simulink model "GVCU_HIL"  (R2026a)
settings: Solver=ode3  StartTime=0  StopTime=2474  FixedStep=0.0002
model workspace (MAT data in the model file):
  CANoelibParameters : object (value not decoded)
values from neighbouring files (symbols this model uses):
  acc_pedal_data = pedal_data.accelerator_pedal_position_t0    [Vehicle_Simulink_init.m]
  acc_pedal_time = pedal_data.t0    [Vehicle_Simulink_init.m]
  brk_pedal_data = brake_pedal_data.shared_brakes_drvrBrkPedlPerc_t0    [Vehicle_Simulink_init.m]
  brk_pedal_time = brake_pedal_data.t0    [Vehicle_Simulink_init.m]
  cycle_len = zeros(1, num_cycles)    [Vehicle_Simulink_init.m]
  cycle_speed_matrix = zeros(max_cycle_len, num_cycles)    [Vehicle_Simulink_init.m]
  cycle_time_matrix = zeros(max_cycle_len, num_cycles)    [Vehicle_Simulink_init.m]
  veh_speed_data = speed_data.shared_dynamicsVso_vehVelLgt_t0    [Vehicle_Simulink_init.m]
  veh_speed_time = speed_data.t0    [Vehicle_Simulink_init.m]
undefined symbols (not defined in the file or in its folder): Active, AuxActive, bat, environment, FL_prs_voltage, FR_prs_voltage, pos, RL_prs_voltage, RR_prs_voltage, tir, veh, VGetRawValueFlag, Voltage, VT2816_1_Ch1, VT2816_1_Ch2, VT2816_1_Ch3, VT2816_1_Ch4, VT2816_3_Ch13, VT2816_3_Ch14, VT7101_1_Out2, VT7820_2_Channel1, VT7820_2_Channel2, VT7820_2_Channel3, VT7820_2_Channel4, VTS
libraries: canoelib x144, autolibsharedcoupling x21, autolibcoupling x9, autolibshared x5, simulink_extras x4, simulink x4, slpidlib x3, autolibshareddiff x3, autolibutils x1, autolibdatasheetbattery x1, autolibmappedmotor x1, sl_discontinuities x1
(part 8 of 9)

== system GVCU_HIL/Vehicle/to grade ==
  In1 : Inport
  Constant : Constant  Value=veh.f + veh.r
  Divide : Product  Inputs=*/
  Gain : Gain  Gain=0.5
  Gain1 : Gain  Gain=0.5
  "Radians to Degrees " : simulink_extras/Transformations/Radians to Degrees
  Selector : Selector  InputPortWidth=4  IndexOptions=Index vector (dialog)  Indices=[1]  OutputSizes=1
  Selector1 : Selector  InputPortWidth=4  IndexOptions=Index vector (dialog)  Indices=[2]  OutputSizes=1
  Selector2 : Selector  InputPortWidth=4  IndexOptions=Index vector (dialog)  Indices=[3]  OutputSizes=1
  Selector3 : Selector  InputPortWidth=4  IndexOptions=Index vector (dialog)  Indices=[4]  OutputSizes=1
  Sum : Sum
  Sum1 : Sum
  Sum2 : Sum  Inputs=+-
  "Tan " : Trigonometry  Operator=asin
  Out1 : Outport
  wires:
  "Radians to Degrees "/1 -> Out1/1
  "Tan "/1 -> "Radians to Degrees "/1
  Divide/1 -> "Tan "/1
  Constant/1 -> Divide/2
  Sum2/1 -> Divide/1
  Gain1/1 -> Sum2/2
  Gain/1 -> Sum2/1
  Sum1/1 -> Gain1/1
  Sum/1 -> Gain/1
  Selector3/1 -> Sum1/2
  Selector2/1 -> Sum1/1
  Selector1/1 -> Sum/2
  Selector/1 -> Sum/1
  In1/1 -> Selector/1, Selector1/1, Selector2/1, Selector3/1

== system GVCU_HIL/Brake_HIL/Simulated GVCU - Steering /Message Output ==
  In1 : Inport
  Bus Selector : BusSelector  OutputSignals=drv_mod,e2e_alive_counter,e2e_checksum,hhc_inhb_req,ieb_chg_mod_req,vdc_perf_mod_req
  S-Function_1 : S-Function  FunctionName=sigout  Parameters=dbName;nodeName;msgName;6;'drv_mod';'e2e_alive_counter';'e2e_checksum';'hhc_inhb_req';'ieb_chg_mod_req';'vdc_perf_mod_req';VGetRawValueFlag(rawValue);'inherited'  SFunctionDeploymentMode=off  EnableBusSupport=off
      settings: AttributesFormatString=drv_mod\ne2e_alive_counter\ne2e_checksum\nhhc_inhb_req\nieb_chg_mod_req\nvdc_perf_mod_req\n
  wires:
  Bus Selector/5 -> S-Function_1/5  "<ieb_chg_mod_req>"
  Bus Selector/4 -> S-Function_1/4  "<hhc_inhb_req>"
  Bus Selector/3 -> S-Function_1/3  "<e2e_checksum>"
  Bus Selector/2 -> S-Function_1/2  "<e2e_alive_counter>"
  Bus Selector/1 -> S-Function_1/1  "<drv_mod>"
  In1/1 -> Bus Selector/1
  Bus Selector/6 -> S-Function_1/6  "<vdc_perf_mod_req>"

== system GVCU_HIL/Brake_HIL/Simulated GVCU - Steering /Message Output1 ==
  In1 : Inport
  Bus Selector : BusSelector  OutputSignals=e2e_alive_counter,e2e_checksum,lat_acc,lat_acc_v,long_acc,long_acc_v,yaw_rate,yaw_rate_v
  S-Function_1 : S-Function  FunctionName=sigout  Parameters=dbName;nodeName;msgName;8;'e2e_alive_counter';'e2e_checksum';'lat_acc';'lat_acc_v';'long_acc';'long_acc_v';'yaw_rate';'yaw_rate_v';VGetRawValueFlag(rawValue);'inherited'  SFunctionDeploymentMode=off  EnableBusSupport=off
      settings: AttributesFormatString=e2e_alive_counter\ne2e_checksum\nlat_acc\nlat_acc_v\nlong_acc\nlong_acc_v\nyaw_rate\nyaw_rate_v\n
  wires:
  Bus Selector/8 -> S-Function_1/8  "<yaw_rate_v>"
  Bus Selector/7 -> S-Function_1/7  "<yaw_rate>"
  Bus Selector/6 -> S-Function_1/6  "<long_acc_v>"
  Bus Selector/5 -> S-Function_1/5  "<long_acc>"
  Bus Selector/4 -> S-Function_1/4  "<lat_acc_v>"
  Bus Selector/3 -> S-Function_1/3  "<lat_acc>"
  Bus Selector/2 -> S-Function_1/2  "<e2e_checksum>"
  Bus Selector/1 -> S-Function_1/1  "<e2e_alive_counter>"
  In1/1 -> Bus Selector/1

== system GVCU_HIL/Brake_HIL/Simulated GVCU - Steering /Message Output2 ==
  In1 : Inport
  Bus Selector : BusSelector  OutputSignals=calibration_sts,e2e_alive_counter,e2e_checksum,steering_wheel_angle,steering_wheel_rot_speed,steering_wheel_sensor_v
  S-Function_1 : S-Function  FunctionName=sigout  Parameters=dbName;nodeName;msgName;6;'calibration_sts';'e2e_alive_counter';'e2e_checksum';'steering_wheel_angle';'steering_wheel_rot_speed';'steering_wheel_sensor_v';VGetRawValueFlag(rawValue);'inherited'  SFunctionDeploymentMode=off  EnableBusSupport=off
      settings: AttributesFormatString=calibration_sts\ne2e_alive_counter\ne2e_checksum\nsteering_wheel_angle\nsteering_wheel_rot_speed\nsteering_wheel_sensor_v\n
  wires:
  Bus Selector/6 -> S-Function_1/6  "<steering_wheel_sensor_v>"
  Bus Selector/5 -> S-Function_1/5  "<steering_wheel_rot_speed>"
  Bus Selector/4 -> S-Function_1/4  "<steering_wheel_angle>"
  Bus Selector/3 -> S-Function_1/3  "<e2e_checksum>"
  Bus Selector/2 -> S-Function_1/2  "<e2e_alive_counter>"
  Bus Selector/1 -> S-Function_1/1  "<calibration_sts>"
  In1/1 -> Bus Selector/1

== system GVCU_HIL/Brake_HIL/Simulated GVCU - Steering /Message Output3 ==
  In1 : Inport
  Bus Selector : BusSelector  OutputSignals=e2e_alive_counter,e2e_checksum,nm_request
  S-Function_1 : S-Function  FunctionName=sigout  Parameters=dbName;nodeName;msgName;3;'e2e_alive_counter';'e2e_checksum';'nm_request';VGetRawValueFlag(rawValue);'inherited'  SFunctionDeploymentMode=off  EnableBusSupport=off
      settings: AttributesFormatString=e2e_alive_counter\ne2e_checksum\nnm_request\n
  wires:
  Bus Selector/3 -> S-Function_1/3  "<nm_request>"
  Bus Selector/2 -> S-Function_1/2  "<e2e_checksum>"
  Bus Selector/1 -> S-Function_1/1  "<e2e_alive_counter>"
  In1/1 -> Bus Selector/1

== system GVCU_HIL/Driver/Driver/Dec_controller ==
  Vel_ref : Inport
  Vel_fdk : Inport  Port=2
  PI Controller : slpidlib/PID Controller  Controller=PI  Form=Parallel  TimeDomain=Discrete-time  UseExternalTs=off  SampleTime=-1  IntegratorMethod=Forward Euler  FilterMethod=Forward Euler  ControllerParametersSource=internal  P=1  I=1  UseKiTs=on  D=0  UseExternalDerivativeSource=off  N=100  UseFilter=on  TunerSelectOption=Transfer Function Based (PID Tuner App)  InitialConditionSource=internal  InitialConditionForIntegrator=0  InitialConditionForFilter=0  DifferentiatorICPrevScaledInput=0  ExternalReset=level  TrackingMode=off  Kt=1  LimitOutput=on  SatLimitsSource=internal  UpperSaturationLimit=50  LowerSaturationLimit=0  LinearizeAsGain=on  AntiWindupMode=clamping  Kb=1  LimitIntegrator=off  UpperIntegratorSaturationLimit=inf  LowerIntegratorSaturationLimit=-inf  RndMeth=Simplest  POutMin=[]  POutMax=[]  IOutMin=[]  IOutMax=[]  DOutMin=[]  DOutMax=[]  NOutMin=[]  NOutMax=[]  SumOutMin=[]  SumOutMax=[]  SaturationOutDataTypeStr=Inherit: Inherit via back propagation  SaturationOutMin=[]  SaturationOutMax=[]  PParamMin=[]  PParamMax=[]  IParamMin=[]  IParamMax=[]  DParamMin=[]  DParamMax=[]  NParamMin=[]  NParamMax=[]  KbParamMin=[]  KbParamMax=[]  KtParamMin=[]  KtParamMax=[]  KbOutMin=[]  KbOutMax=[]  KtOutMin=[]  KtOutMax=[]  IntegratorOutMin=[]  IntegratorOutMax=[]  FilterOutMin=[]  FilterOutMax=[]  SumI1OutMin=[]  SumI1OutMax=[]  SumI2OutMin=[]  SumI2OutMax=[]  SumI3OutMin=[]  SumI3OutMax=[]  SumI4OutMin=[]  SumI4OutMax=[]  SumDOutMin=[]  SumDOutMax=[]  DifferentiatorOutMin=[]  DifferentiatorOutMax=[]  FilterDiffOutCoefMin=[]  FilterDiffOutCoefMax=[]  ReciprocalOutMin=[]  ReciprocalOutMax=[]  SumDenOutMin=[]  SumDenOutMax=[]  SumNumOutMin=[]  SumNumOutMax=[]  DivideOutMin=[]  DivideOutMax=[]  UdiffTsProdOutMin=[]  UdiffTsProdOutMax=[]  NTsProdOutMin=[]  NTsProdOutMax=[]  UintegralTsProdOutMin=[]  UintegralTsProdOutMax=[]  UngainTsProdOutMin=[]  UngainTsProdOutMax=[]  ClampingZeroOutDataTypeStr=Inherit: Inherit via back propagation  ClampingZeroOutMin=[]  ClampingZeroOutMax=[]  FilterDenConstantOutDataTypeStr=Inherit: Inherit via back propagation  FilterDenConstantOutMin=[]  FilterDenConstantOutMax=[]  PCopyOutDataTypeStr=Inherit: Inherit via back propagation  PCopyOutMin=[]  PCopyOutMax=[]  NCopyOutDataTypeStr=Inherit: Inherit via back propagation  NCopyOutMin=[]  NCopyOutMax=[]  IntegratorContinuousStateAttributes=''  IntegratorStateMustResolveToSignalObject=off  IntegratorRTWStateStorageClass=Auto  FilterContinuousStateAttributes=''  FilterStateMustResolveToSignalObject=off  FilterRTWStateStorageClass=Auto  ParallelPVariant=InternalParameters  IdealPVariant=Disabled  IVariant=InternalParameters  DVariant=Disabled  IntegratorVariant=Discrete  SatVariant=Enabled  AWVariant=DiscClampingParallel  PCopyVariant=Disabled  TRVariant=Disabled  FdbkBlocksVariant=Forward  IdealPFdbkVariant=Disabled  SatFdbkVariant=Disabled  DerivativeFilterVariant=Disabled  NVariant=Disabled  NCopyVariant=Disabled_SignalSpec  FilterICVariant=Disabled  IntegratorICVariant=InternalICs  ExternalResetVariant=ExternalReset  TRSumVariant=Passthrough  SumFdbkVariant=Disabled  SumVariant=Sum_PI  TsampFilterVariant=InternalTs  TsampNgainVariant=Passthrough  TsampIntegralVariant=Disabled_SignalSpec  ExternalSaturationOutDataTypeStr=Inherit: Same as second input  DerivativeSourceVariant=Disabled  PreIntVariant=InternalPreInt
      settings: LibrarySourceBlock=mcbhdllib/Controls/Controllers/PI Controller
  Relay : Relay  OnSwitchValue=10  OffSwitchValue=1
  Subtract : Sum  Inputs=+-
  Dec_cmd : Outport
  wires:
  Vel_ref/1 -> Subtract/2
  Vel_fdk/1 -> Subtract/1
  PI Controller/1 -> Dec_cmd/1
  Subtract/1 -> PI Controller/1, Relay/1
  Relay/1 -> PI Controller/2

== system GVCU_HIL/Driver/Driver/LPF ==
  u : Inport
  Divide : Product  Inputs=/
  Error LPF : autolibutils/Cont LPF Dyn  aMode=aMode  dataType=off
  tauerr : Constant  Value=0.03  SampleTime=-1
  y : Outport  VectorParamsAs1DForOutWhenUnconnected=off
  wires:
  Error LPF/1 -> y/1
  Divide/1 -> Error LPF/2
  tauerr/1 -> Divide/1
  u/1 -> Error LPF/1

== system GVCU_HIL/GVCU - HiL/Commented messages/Message Output12 ==
  In1 : Inport
  Bus Selector : BusSelector  OutputSignals=e2e_alive_counter_disabled,e2e_checksum_disabled,e_motor_pump_fault,e_motor_pump_power_on,e_motor_pump_speed,e_motor_pump_warning,front_left_fan_fault,front_left_fan_power_on,front_left_fan_speed,front_left_fan_warning,hv_bat_pump_fault,hv_bat_pump_power_on,hv_bat_pump_speed,hv_bat_pump_warning
  S-Function_1 : S-Function  FunctionName=sigout  Parameters=dbName;nodeName;msgName;14;'e2e_alive_counter_disabled';'e2e_checksum_disabled';'e_motor_pump_fault';'e_motor_pump_power_on';'e_motor_pump_speed';'e_motor_pump_warning';'front_left_fan_fault';'front_left_fan_power_on';'front_left_fan_speed';'front_left_fan_warning';'hv_bat_pump_fault';'hv_bat_pump_power_on';'hv_bat_pump_speed';'hv_bat_pump_warning';VGetRawValueFlag(rawValue);'inherited'  SFunctionDeploymentMode=off  EnableBusSupport=off
      settings: AttributesFormatString=e2e_alive_counter_disabled\ne2e_checksum_disabled\ne_motor_pump_fault\ne_motor_pump_power_on\ne_motor_pump_speed\ne_motor_pump_warning\nfront_left_fan_fault\nfront_left_fan_power_on\nfront_left_fan_speed\nfront_left_fan_warning\nhv_bat_pump_fault\nhv_bat_pump_power_on\nhv_bat_pump_speed\nhv_bat_pump_warning\n
  wires:
  In1/1 -> Bus Selector/1
  Bus Selector/1 -> S-Function_1/1  "<e2e_alive_counter_disabled>"
  Bus Selector/2 -> S-Function_1/2  "<e2e_checksum_disabled>"
  Bus Selector/3 -> S-Function_1/3  "<e_motor_pump_fault>"
  Bus Selector/4 -> S-Function_1/4  "<e_motor_pump_power_on>"
  Bus Selector/5 -> S-Function_1/5  "<e_motor_pump_speed>"
  Bus Selector/6 -> S-Function_1/6  "<e_motor_pump_warning>"
  Bus Selector/7 -> S-Function_1/7  "<front_left_fan_fault>"
  Bus Selector/8 -> S-Function_1/8  "<front_left_fan_power_on>"
  Bus Selector/9 -> S-Function_1/9  "<front_left_fan_speed>"
  Bus Selector/10 -> S-Function_1/10  "<front_left_fan_warning>"
  Bus Selector/11 -> S-Function_1/11  "<hv_bat_pump_fault>"
  Bus Selector/12 -> S-Function_1/12  "<hv_bat_pump_power_on>"
  Bus Selector/13 -> S-Function_1/13  "<hv_bat_pump_speed>"
  Bus Selector/14 -> S-Function_1/14  "<hv_bat_pump_warning>"

== system GVCU_HIL/GVCU - HiL/Commented messages/Message Output13 ==
  In1 : Inport
  Bus Selector : BusSelector  OutputSignals=e2e_alive_counter_disabled,e2e_checksum_disabled,inverter_pump_fault,inverter_pump_power_on,inverter_pump_speed,inverter_pump_warning
  S-Function_1 : S-Function  FunctionName=sigout  Parameters=dbName;nodeName;msgName;6;'e2e_alive_counter_disabled';'e2e_checksum_disabled';'inverter_pump_fault';'inverter_pump_power_on';'inverter_pump_speed';'inverter_pump_warning';VGetRawValueFlag(rawValue);'inherited'  SFunctionDeploymentMode=off  EnableBusSupport=off
      settings: AttributesFormatString=e2e_alive_counter_disabled\ne2e_checksum_disabled\ninverter_pump_fault\ninverter_pump_power_on\ninverter_pump_speed\ninverter_pump_warning\n
  wires:
  In1/1 -> Bus Selector/1
  Bus Selector/1 -> S-Function_1/1  "<e2e_alive_counter_disabled>"
  Bus Selector/2 -> S-Function_1/2  "<e2e_checksum_disabled>"
  Bus Selector/3 -> S-Function_1/3  "<inverter_pump_fault>"
  Bus Selector/4 -> S-Function_1/4  "<inverter_pump_power_on>"
  Bus Selector/5 -> S-Function_1/5  "<inverter_pump_speed>"
  Bus Selector/6 -> S-Function_1/6  "<inverter_pump_warning>"

== system GVCU_HIL/GVCU - HiL/Commented messages/Message Output14 ==
  In1 : Inport
  Bus Selector : BusSelector  OutputSignals=u_lift_cyl_fl,u_lift_cyl_fr,u_wishbone_angle_fl,u_wishbone_angle_fr
  S-Function_1 : S-Function  FunctionName=sigout  Parameters=dbName;nodeName;msgName;4;'u_lift_cyl_fl';'u_lift_cyl_fr';'u_wishbone_angle_fl';'u_wishbone_angle_fr';VGetRawValueFlag(rawValue);'inherited'  SFunctionDeploymentMode=off  EnableBusSupport=off
      settings: AttributesFormatString=u_lift_cyl_fl\nu_lift_cyl_fr\nu_wishbone_angle_fl\nu_wishbone_angle_fr\n
  wires:
  In1/1 -> Bus Selector/1
  Bus Selector/1 -> S-Function_1/1  "<u_lift_cyl_fl>"
  Bus Selector/2 -> S-Function_1/2  "<u_lift_cyl_fr>"
  Bus Selector/3 -> S-Function_1/3  "<u_wishbone_angle_fl>"
  Bus Selector/4 -> S-Function_1/4  "<u_wishbone_angle_fr>"

== system GVCU_HIL/GVCU - HiL/Commented messages/Message Output15 ==
  In1 : Inport
  Bus Selector : BusSelector  OutputSignals=actv_re,snsr_data_rcl,snsr_data_rcr,snsr_data_rl,snsr_data_rll,snsr_data_rr,snsr_data_rrl,snsr_st_rcl,snsr_st_rcr,snsr_st_rl,snsr_st_rll,snsr_st_rr,snsr_st_rrl
  S-Function_1 : S-Function  FunctionName=sigout  Parameters=dbName;nodeName;msgName;13;'actv_re';'snsr_data_rcl';'snsr_data_rcr';'snsr_data_rl';'snsr_data_rll';'snsr_data_rr';'snsr_data_rrl';'snsr_st_rcl';'snsr_st_rcr';'snsr_st_rl';'snsr_st_rll';'snsr_st_rr';'snsr_st_rrl';VGetRawValueFlag(rawValue);'inherited'  SFunctionDeploymentMode=off  EnableBusSupport=off
      settings: AttributesFormatString=actv_re\nsnsr_data_rcl\nsnsr_data_rcr\nsnsr_data_rl\nsnsr_data_rll\nsnsr_data_rr\nsnsr_data_rrl\nsnsr_st_rcl\nsnsr_st_rcr\nsnsr_st_rl\nsnsr_st_rll\nsnsr_st_rr\nsnsr_st_rrl\n
  wires:
  In1/1 -> Bus Selector/1
  Bus Selector/1 -> S-Function_1/1  "<actv_re>"
  Bus Selector/2 -> S-Function_1/2  "<snsr_data_rcl>"
  Bus Selector/3 -> S-Function_1/3  "<snsr_data_rcr>"
  Bus Selector/4 -> S-Function_1/4  "<snsr_data_rl>"
  Bus Selector/5 -> S-Function_1/5  "<snsr_data_rll>"
  Bus Selector/6 -> S-Function_1/6  "<snsr_data_rr>"
  Bus Selector/7 -> S-Function_1/7  "<snsr_data_rrl>"
  Bus Selector/8 -> S-Function_1/8  "<snsr_st_rcl>"
  Bus Selector/9 -> S-Function_1/9  "<snsr_st_rcr>"
  Bus Selector/10 -> S-Function_1/10  "<snsr_st_rl>"
  Bus Selector/11 -> S-Function_1/11  "<snsr_st_rll>"
  Bus Selector/12 -> S-Function_1/12  "<snsr_st_rr>"
  Bus Selector/13 -> S-Function_1/13  "<snsr_st_rrl>"

== system GVCU_HIL/GVCU - HiL/Commented messages/Message Output16 ==
  In1 : Inport
  Bus Selector : BusSelector  OutputSignals=actv_frnt,snsr_data_fcl,snsr_data_fcr,snsr_data_fl,snsr_data_fll,snsr_data_fr,snsr_data_frl,snsr_st_fcl,snsr_st_fcr,snsr_st_fl,snsr_st_fll,snsr_st_fr,snsr_st_frl
  S-Function_1 : S-Function  FunctionName=sigout  Parameters=dbName;nodeName;msgName;13;'actv_frnt';'snsr_data_fcl';'snsr_data_fcr';'snsr_data_fl';'snsr_data_fll';'snsr_data_fr';'snsr_data_frl';'snsr_st_fcl';'snsr_st_fcr';'snsr_st_fl';'snsr_st_fll';'snsr_st_fr';'snsr_st_frl';VGetRawValueFlag(rawValue);'inherited'  SFunctionDeploymentMode=off  EnableBusSupport=off
      settings: AttributesFormatString=actv_frnt\nsnsr_data_fcl\nsnsr_data_fcr\nsnsr_data_fl\nsnsr_data_fll\nsnsr_data_fr\nsnsr_data_frl\nsnsr_st_fcl\nsnsr_st_fcr\nsnsr_st_fl\nsnsr_st_fll\nsnsr_st_fr\nsnsr_st_frl\n
  wires:
  In1/1 -> Bus Selector/1
  Bus Selector/1 -> S-Function_1/1  "<actv_frnt>"
  Bus Selector/2 -> S-Function_1/2  "<snsr_data_fcl>"
  Bus Selector/3 -> S-Function_1/3  "<snsr_data_fcr>"
  Bus Selector/4 -> S-Function_1/4  "<snsr_data_fl>"
  Bus Selector/5 -> S-Function_1/5  "<snsr_data_fll>"
  Bus Selector/6 -> S-Function_1/6  "<snsr_data_fr>"
  Bus Selector/7 -> S-Function_1/7  "<snsr_data_frl>"
  Bus Selector/8 -> S-Function_1/8  "<snsr_st_fcl>"
  Bus Selector/9 -> S-Function_1/9  "<snsr_st_fcr>"
  Bus Selector/10 -> S-Function_1/10  "<snsr_st_fl>"
  Bus Selector/11 -> S-Function_1/11  "<snsr_st_fll>"
  Bus Selector/12 -> S-Function_1/12  "<snsr_st_fr>"
  Bus Selector/13 -> S-Function_1/13  "<snsr_st_frl>"

== system GVCU_HIL/GVCU - HiL/Commented messages/Message Output2 ==
  In1 : Inport
  Bus Selector : BusSelector  OutputSignals=e2e_alive_counter_disabled,e2e_checksum_disabled,front_center_left_fan_fault,front_center_left_fan_power_on,front_center_left_fan_speed,front_center_left_fan_warning,front_center_right_fan_fault,front_center_right_fan_power_on,front_center_right_fan_speed,front_center_right_fan_warning,front_right_fan_fault,front_right_fan_power_on,front_right_fan_speed,front_right_fan_warning
  S-Function_1 : S-Function  FunctionName=sigout  Parameters=dbName;nodeName;msgName;14;'e2e_alive_counter_disabled';'e2e_checksum_disabled';'front_center_left_fan_fault';'front_center_left_fan_power_on';'front_center_left_fan_speed';'front_center_left_fan_warning';'front_center_right_fan_fault';'front_center_right_fan_power_on';'front_center_right_fan_speed';'front_center_right_fan_warning';'front_right_fan_fault';'front_right_fan_power_on';'front_right_fan_speed';'front_right_fan_warning';VGetRawValueFlag(rawValue);'inherited'  SFunctionDeploymentMode=off  EnableBusSupport=off
      settings: AttributesFormatString=e2e_alive_counter_disabled\ne2e_checksum_disabled\nfront_center_left_fan_fault\nfront_center_left_fan_power_on\nfront_center_left_fan_speed\nfront_center_left_fan_warning\nfront_center_right_fan_fault\nfront_center_right_fan_power_on\nfront_center_right_fan_speed\nfront_center_right_fan_warning\nfront_right_fan_fault\nfront_right_fan_power_on\nfront_right_fan_speed\nfront_right_fan_warning\n
  wires:
  In1/1 -> Bus Selector/1
  Bus Selector/1 -> S-Function_1/1  "<e2e_alive_counter_disabled>"
  Bus Selector/2 -> S-Function_1/2  "<e2e_checksum_disabled>"
  Bus Selector/3 -> S-Function_1/3  "<front_center_left_fan_fault>"
  Bus Selector/4 -> S-Function_1/4  "<front_center_left_fan_power_on>"
  Bus Selector/5 -> S-Function_1/5  "<front_center_left_fan_speed>"
  Bus Selector/6 -> S-Function_1/6  "<front_center_left_fan_warning>"
  Bus Selector/7 -> S-Function_1/7  "<front_center_right_fan_fault>"
  Bus Selector/8 -> S-Function_1/8  "<front_center_right_fan_power_on>"
  Bus Selector/9 -> S-Function_1/9  "<front_center_right_fan_speed>"
  Bus Selector/10 -> S-Function_1/10  "<front_center_right_fan_warning>"
  Bus Selector/11 -> S-Function_1/11  "<front_right_fan_fault>"
  Bus Selector/12 -> S-Function_1/12  "<front_right_fan_power_on>"
  Bus Selector/13 -> S-Function_1/13  "<front_right_fan_speed>"
  Bus Selector/14 -> S-Function_1/14  "<front_right_fan_warning>"

== system GVCU_HIL/GVCU - HiL/Commented messages/Message Output20 ==
  In1 : Inport
  Bus Selector : BusSelector  OutputSignals=E2eAliveCounter_Disable,E2eChecksum_Disable,acc_dft_actv_st,acc_dft_dist_lvl,auto_upsh_btn_st,drv_cfg_req,drv_st,esp_st_req,forced_chrg_btn_st,lift_mod_btn_st,man_mod_btn_st,suppg_mod_req,tire_mdl_req
  S-Function_1 : S-Function  FunctionName=sigout  Parameters=dbName;nodeName;msgName;13;'E2eAliveCounter_Disable';'E2eChecksum_Disable';'acc_dft_actv_st';'acc_dft_dist_lvl';'auto_upsh_btn_st';'drv_cfg_req';'drv_mod_req';'esp_st_req';'forced_chrg_btn_st';'lift_mod_btn_st';'man_mod_btn_st';'suppg_mod_req';'tire_mdl_req';VGetRawValueFlag(rawValue);'inherited'  SFunctionDeploymentMode=off  EnableBusSupport=off
      settings: AttributesFormatString=E2eAliveCounter_Disable\nE2eChecksum_Disable\nacc_dft_actv_st\nacc_dft_dist_lvl\nauto_upsh_btn_st\ndrv_cfg_req\ndrv_mod_req\nesp_st_req\nforced_chrg_btn_st\nlift_mod_btn_st\nman_mod_btn_st\nsuppg_mod_req\ntire_mdl_req\n
  wires:
  In1/1 -> Bus Selector/1
  Bus Selector/1 -> S-Function_1/1  "<E2eAliveCounter_Disable>"
  Bus Selector/2 -> S-Function_1/2  "<E2eChecksum_Disable>"
  Bus Selector/3 -> S-Function_1/3  "<acc_dft_actv_st>"
  Bus Selector/4 -> S-Function_1/4  "<acc_dft_dist_lvl>"
  Bus Selector/5 -> S-Function_1/5  "<auto_upsh_btn_st>"
  ? -> S-Function_1/6  "<drift_mod_st_req>"
  Bus Selector/6 -> S-Function_1/7  "<drv_cfg_req>"
  Bus Selector/7 -> S-Function_1/8  "<drv_st>"
  Bus Selector/8 -> S-Function_1/9  "<esp_st_req>"
  Bus Selector/9 -> S-Function_1/10  "<forced_chrg_btn_st>"
  Bus Selector/10 -> S-Function_1/11  "<lift_mod_btn_st>"
  Bus Selector/11 -> S-Function_1/12  "<man_mod_btn_st>"
  Bus Selector/13 -> S-Function_1/13  "<tire_mdl_req>"

== system GVCU_HIL/GVCU - HiL/Commented messages/Message Output4 ==
  In1 : Inport
  Bus Selector : BusSelector  OutputSignals=CrashSeverity,DriverSideCrash,E2eAliveCounter,E2eChecksum,FrontCrash,PassSideCrash,RearCrash,RolloverCrash
  S-Function_1 : S-Function  FunctionName=sigout  Parameters=dbName;nodeName;msgName;8;'CrashSeverity';'DriverSideCrash';'E2eAliveCounter';'E2eChecksum';'FrontCrash';'PassSideCrash';'RearCrash';'RolloverCrash';VGetRawValueFlag(rawValue);'inherited'  SFunctionDeploymentMode=off  EnableBusSupport=off
      settings: AttributesFormatString=CrashSeverity\nDriverSideCrash\nE2eAliveCounter\nE2eChecksum\nFrontCrash\nPassSideCrash\nRearCrash\nRolloverCrash\n
  wires:
  In1/1 -> Bus Selector/1
  Bus Selector/1 -> S-Function_1/1  "<CrashSeverity>"
  Bus Selector/2 -> S-Function_1/2  "<DriverSideCrash>"
  Bus Selector/3 -> S-Function_1/3  "<E2eAliveCounter>"
  Bus Selector/4 -> S-Function_1/4  "<E2eChecksum>"
  Bus Selector/5 -> S-Function_1/5  "<FrontCrash>"
  Bus Selector/6 -> S-Function_1/6  "<PassSideCrash>"
  Bus Selector/7 -> S-Function_1/7  "<RearCrash>"
  Bus Selector/8 -> S-Function_1/8  "<RolloverCrash>"

== system GVCU_HIL/GVCU - HiL/Commented messages/Message Output5 ==
  In1 : Inport
  Bus Selector : BusSelector  OutputSignals=CrashOutput,E2eAliveCounter,E2eChecksum
  S-Function_1 : S-Function  FunctionName=sigout  Parameters=dbName;nodeName;msgName;3;'CrashOutput';'E2eAliveCounter';'E2eChecksum';VGetRawValueFlag(rawValue);'inherited'  SFunctionDeploymentMode=off  EnableBusSupport=off
      settings: AttributesFormatString=CrashOutput\nE2eAliveCounter\nE2eChecksum\n
  wires:
  In1/1 -> Bus Selector/1
  Bus Selector/1 -> S-Function_1/1  "<CrashOutput>"
  Bus Selector/2 -> S-Function_1/2  "<E2eAliveCounter>"
  Bus Selector/3 -> S-Function_1/3  "<E2eChecksum>"

== system GVCU_HIL/GVCU - HiL/Commented messages/Message Output6 ==
  In1 : Inport
  Bus Selector : BusSelector  OutputSignals=center_left_fan_bat_vltg,center_left_fan_can_collision,center_left_fan_can_watchdog,center_left_fan_motor_stall,center_left_fan_over_crnt,center_left_fan_over_pwr,center_left_fan_over_temp,center_right_fan_bat_vltg,center_right_fan_can_collision,center_right_fan_can_watchdog,center_right_fan_motor_stall,center_right_fan_over_crnt,center_right_fan_over_pwr,center_right_fan_over_temp,e_mot_pump_comm_fault,e_mot_pump_int_op_fault,e_mot_pump_over_crnt,e_mot_pump_over_temp,e_mot_pump_vltg_err,front_left_fan_bat_vltg,front_left_fan_can_collision,front_left_fan_can_watchdog,front_left_fan_motor_stall,front_left_fan_over_crnt,front_left_fan_over_pwr,front_left_fan_over_temp,front_right_fan_bat_vltg,front_right_fan_can_collision,front_right_fan_can_watchdog,front_right_fan_motor_stall,front_right_fan_over_crnt,front_right_fan_over_pwr,front_right_fan_over_temp,hv_bat_pump_bat_vltg,hv_bat_pump_can_collision,hv_bat_pump_can_watchdog,hv_bat_pump_motor_stall,hv_bat_pump_over_crnt,hv_bat_pump_over_pwr,hv_bat_pump_over_temp,inverter_pump_bat_vltg,inverter_pump_can_collision,inverter_pump_can_watchdog,inverter_pump_motor_stall,inverter_pump_over_crnt,inverter_pump_over_pwr,inverter_pump_over_temp
  S-Function_1 : S-Function  FunctionName=sigout  Parameters=dbName;nodeName;msgName;47;'center_left_fan_bat_vltg';'center_left_fan_can_collision';'center_left_fan_can_watchdog';'center_left_fan_motor_stall';'center_left_fan_over_crnt';'center_left_fan_over_pwr';'center_left_fan_over_temp';'center_right_fan_bat_vltg';'center_right_fan_can_collision';'center_right_fan_can_watchdog';'center_right_fan_motor_stall';'center_right_fan_over_crnt';'center_right_fan_over_pwr';'center_right_fan_over_temp';'e_mot_pump_comm_fault';'e_mot_pump_int_op_fault';'e_mot_pump_over_crnt';'e_mot_pump_over_temp';'e_mot_pump_vltg_err';'front_left_fan_bat_vltg';'front_left_fan_can_collision';'front_left_fan_can_watchdog';'front_left_fan_motor_stall';'front_left_fan_over_crnt';'front_left_fan_over_pwr';'front_left_fan_over_temp';'front_right_fan_bat_vltg';'front_right_fan_can_collision';'front_right_fan_can_watchdog';'front_right_fan_motor_stall';'front_right_fan_over_crnt';'front_right_fan_over_pwr';'front_right_fan_over_temp';'hv_bat_pump_bat_vltg';'hv_bat_pump_can_collision';'hv_bat_pump_can_watchdog';'hv_bat_pump_motor_stall';'hv_bat_pump_over_crnt';'hv_bat_pump_over_pwr';'hv_bat_pump_over_temp';'inverter_pump_bat_vltg';'inverter_pump_can_collision';'inverter_pump_can_watchdog';'inverter_pump_motor_stall';'inverter_pump_over_crnt';'inverter_pump_over_pwr';'inverter_pump_over_temp';VGetRawValueFlag(rawValue);'inherited'  SFunctionDeploymentMode=off  EnableBusSupport=off
      settings: AttributesFormatString=center_left_fan_bat_vltg\ncenter_left_fan_can_collision\ncenter_left_fan_can_watchdog\ncenter_left_fan_motor_stall\ncenter_left_fan_over_crnt\ncenter_left_fan_over_pwr\ncenter_left_fan_over_temp\ncenter_right_fan_bat_vltg\ncenter_right_fan_can_collision\ncenter_right_fan_can_watchdog\ncenter_right_fan_motor_stall\ncenter_right_fan_over_crnt\ncenter_right_fan_over_pwr\ncenter_right_fan_over_temp\ne_mot_pump_comm_fault\ne_mot_pump_int_op_fault\ne_mot_pump_over_crnt\ne_mot_pump_over_temp\ne_mot_pump_vltg_err\nfront_left_fan_bat_vltg\nfront_left_fan_can_collision\nfront_left_fan_can_watchdog\nfront_left_fan_motor_stall\nfront_left_fan_over_crnt\nfront_left_fan_over_pwr\nfront_left_fan_over_temp\nfront_right_fan_bat_vltg\nfront_right_fan_can_collision\nfront_right_fan_can_watchdog\nfront_right_fan_motor_stall\nfront_right_fan_over_crnt\nfront_right_fan_over_pwr\nfront_right_fan_over_temp\nhv_bat_pump_bat_vltg\nhv_bat_pump_can_collision\nhv_bat_pump_can_watchdog\nhv_bat_pump_motor_stall\nhv_bat_pump_over_crnt\nhv_bat_pump_over_pwr\nhv_bat_pump_over_temp\ninverter_pump_bat_vltg\ninverter_pump_can_collision\ninverter_pump_can_watchdog\ninverter_pump_motor_stall\ninverter_pump_over_crnt\ninverter_pump_over_pwr\ninverter_pump_over_temp\n
  wires:
  In1/1 -> Bus Selector/1
  Bus Selector/1 -> S-Function_1/1  "<center_left_fan_bat_vltg>"
  Bus Selector/2 -> S-Function_1/2  "<center_left_fan_can_collision>"
  Bus Selector/3 -> S-Function_1/3  "<center_left_fan_can_watchdog>"
  Bus Selector/4 -> S-Function_1/4  "<center_left_fan_motor_stall>"
  Bus Selector/5 -> S-Function_1/5  "<center_left_fan_over_crnt>"
  Bus Selector/6 -> S-Function_1/6  "<center_left_fan_over_pwr>"
  Bus Selector/7 -> S-Function_1/7  "<center_left_fan_over_temp>"
  Bus Selector/8 -> S-Function_1/8  "<center_right_fan_bat_vltg>"
  Bus Selector/9 -> S-Function_1/9  "<center_right_fan_can_collision>"
  Bus Selector/10 -> S-Function_1/10  "<center_right_fan_can_watchdog>"
  Bus Selector/11 -> S-Function_1/11  "<center_right_fan_motor_stall>"
  Bus Selector/12 -> S-Function_1/12  "<center_right_fan_over_crnt>"
  Bus Selector/13 -> S-Function_1/13  "<center_right_fan_over_pwr>"
  Bus Selector/14 -> S-Function_1/14  "<center_right_fan_over_temp>"
  Bus Selector/15 -> S-Function_1/15  "<e_mot_pump_comm_fault>"
  Bus Selector/16 -> S-Function_1/16  "<e_mot_pump_int_op_fault>"
  Bus Selector/17 -> S-Function_1/17  "<e_mot_pump_over_crnt>"
  Bus Selector/18 -> S-Function_1/18  "<e_mot_pump_over_temp>"
  Bus Selector/19 -> S-Function_1/19  "<e_mot_pump_vltg_err>"
  Bus Selector/20 -> S-Function_1/20  "<front_left_fan_bat_vltg>"
  Bus Selector/21 -> S-Function_1/21  "<front_left_fan_can_collision>"
  Bus Selector/22 -> S-Function_1/22  "<front_left_fan_can_watchdog>"
  Bus Selector/23 -> S-Function_1/23  "<front_left_fan_motor_stall>"
  Bus Selector/24 -> S-Function_1/24  "<front_left_fan_over_crnt>"
  Bus Selector/25 -> S-Function_1/25  "<front_left_fan_over_pwr>"
  Bus Selector/26 -> S-Function_1/26  "<front_left_fan_over_temp>"
  Bus Selector/27 -> S-Function_1/27  "<front_right_fan_bat_vltg>"
  Bus Selector/28 -> S-Function_1/28  "<front_right_fan_can_collision>"
  Bus Selector/29 -> S-Function_1/29  "<front_right_fan_can_watchdog>"
  Bus Selector/30 -> S-Function_1/30  "<front_right_fan_motor_stall>"
  Bus Selector/31 -> S-Function_1/31  "<front_right_fan_over_crnt>"
  Bus Selector/32 -> S-Function_1/32  "<front_right_fan_over_pwr>"
  Bus Selector/33 -> S-Function_1/33  "<front_right_fan_over_temp>"
  Bus Selector/34 -> S-Function_1/34  "<hv_bat_pump_bat_vltg>"
  Bus Selector/35 -> S-Function_1/35  "<hv_bat_pump_can_collision>"
  Bus Selector/36 -> S-Function_1/36  "<hv_bat_pump_can_watchdog>"
  Bus Selector/37 -> S-Function_1/37  "<hv_bat_pump_motor_stall>"
  Bus Selector/38 -> S-Function_1/38  "<hv_bat_pump_over_crnt>"
  Bus Selector/39 -> S-Function_1/39  "<hv_bat_pump_over_pwr>"
  Bus Selector/40 -> S-Function_1/40  "<hv_bat_pump_over_temp>"
  Bus Selector/41 -> S-Function_1/41  "<inverter_pump_bat_vltg>"
  Bus Selector/42 -> S-Function_1/42  "<inverter_pump_can_collision>"
  Bus Selector/43 -> S-Function_1/43  "<inverter_pump_can_watchdog>"
  Bus Selector/44 -> S-Function_1/44  "<inverter_pump_motor_stall>"
  Bus Selector/45 -> S-Function_1/45  "<inverter_pump_over_crnt>"
  Bus Selector/46 -> S-Function_1/46  "<inverter_pump_over_pwr>"
  Bus Selector/47 -> S-Function_1/47  "<inverter_pump_over_temp>"

== system GVCU_HIL/GVCU - HiL/Commented messages/Message Output9 ==
  In1 : Inport
  Bus Selector : BusSelector  OutputSignals=charge_current,charge_port_status,charge_voltage,charging_mode,e2e_alive_counter_disabled,e2e_checksum_disabled,evcc_status,inlet_motor_status,obc_fan_req,obc_pump_req,obc_status
  S-Function_1 : S-Function  FunctionName=sigout  Parameters=dbName;nodeName;msgName;11;'charge_current';'charge_port_status';'charge_voltage';'charging_mode';'e2e_alive_counter_disabled';'e2e_checksum_disabled';'evcc_status';'inlet_motor_status';'obc_fan_req';'obc_pump_req';'obc_status';VGetRawValueFlag(rawValue);'inherited'  SFunctionDeploymentMode=off  EnableBusSupport=off
      settings: AttributesFormatString=charge_current\ncharge_port_status\ncharge_voltage\ncharging_mode\ne2e_alive_counter_disabled\ne2e_checksum_disabled\nevcc_status\ninlet_motor_status\nobc_fan_req\nobc_pump_req\nobc_status\n
  wires:
  In1/1 -> Bus Selector/1
  Bus Selector/1 -> S-Function_1/1  "<charge_current>"
  Bus Selector/2 -> S-Function_1/2  "<charge_port_status>"
  Bus Selector/3 -> S-Function_1/3  "<charge_voltage>"
  Bus Selector/4 -> S-Function_1/4  "<charging_mode>"
  Bus Selector/5 -> S-Function_1/5  "<e2e_alive_counter_disabled>"
  Bus Selector/6 -> S-Function_1/6  "<e2e_checksum_disabled>"
  Bus Selector/7 -> S-Function_1/7  "<evcc_status>"
  Bus Selector/8 -> S-Function_1/8  "<inlet_motor_status>"
  Bus Selector/9 -> S-Function_1/9  "<obc_fan_req>"
  Bus Selector/10 -> S-Function_1/10  "<obc_pump_req>"
  Bus Selector/11 -> S-Function_1/11  "<obc_status>"

== system GVCU_HIL/Powertrain (EV)/AWD_Powertrain1/Central axle ==
  Rear_axle_speed : Inport
  Tosional_rear_c : Inport  Port=2
  Central_Clutch : autolibcoupling/Disc Clutch  port_config=Simulink  Reff=.091/2  Ndisk=9  Aeff=0.006283185  Peng=320000  Jin=.1  Jout=.1  muk=.088  mus=.089  bin=.001  bout=.001  win_o=pos.xdot_0/veh.TyreLoadedRadius_F*veh.BevelGear_F  wout_o=pos.xdot_0/veh.TyreLoadedRadius_F*veh.BevelGear_F  tauC=.01  InitiallyLocked=off  maxAbsSpd=3000  blkID=1
  FR1 : autolibsharedcoupling/Torsional Compliance  port_config=Simulink  extInfo=off  k=5e4  b=4e2  theta_o=0  domega_o=0  omega_c=3000  blkID=0  aMode=1
  FR2 : autolibsharedcoupling/Torsional Compliance  port_config=Simulink  extInfo=off  k=5e4  b=4e2  theta_o=0  domega_o=0  omega_c=3000  blkID=0  aMode=1
  Gain1 : Gain  Gain=1/0.93
  Terminator : Terminator
  drop gear + omega_to_rpm_central : Gain  Gain=0.92 *30/pi
  Prop_shaft_trq : Outport
  Central_axle_trq : Outport  Port=2
  tag scope: third_shaft_spd=global
  wires:
  Central_Clutch/1 -> Terminator/1
  [Center_prs] -> Central_Clutch/1
  FR2/2 -> Central_Clutch/2
  Gain1/1 -> Prop_shaft_trq/1
  FR1/2 -> Gain1/1
  Tosional_rear_c/1 -> drop gear + omega_to_rpm_central/1, FR1/2
  FR2/1 -> Central_axle_trq/1
  FR1/1 -> Central_Clutch/3
  Central_Clutch/3 -> FR1/1
  Central_Clutch/2 -> FR2/2  "FrontSpd"
  Rear_axle_speed/1 -> FR2/1
  drop gear + omega_to_rpm_central/1 -> [third_shaft_spd]  "Front_axle_freq"

== system GVCU_HIL/Powertrain (EV)/AWD_Powertrain1/Front Axle ==
  AxlSpd : Inport
  Veh : Inport  Port=2
  Bus Selector : BusSelector  OutputSignals=Wheels.Omega
  Demux : Demux
  FL : autolibsharedcoupling/Torsional Compliance  port_config=Simulink  extInfo=off  k=5e4  b=4e2  theta_o=0  domega_o=0  omega_c=3000  blkID=0  aMode=1
  FL_Clutch : autolibcoupling/Disc Clutch  port_config=Simulink  Reff=.091/2  Ndisk=9  Aeff=0.006283185  Peng=320000  Jin=.1  Jout=.1  muk=.088  mus=.089  bin=.001  bout=.001  win_o=pos.xdot_0/veh.TyreLoadedRadius_F  wout_o=pos.xdot_0/veh.TyreLoadedRadius_F  tauC=1  InitiallyLocked=off  maxAbsSpd=3000  blkID=1
  FR : autolibsharedcoupling/Torsional Compliance  port_config=Simulink  extInfo=off  k=5e4  b=4e2  theta_o=0  domega_o=0  omega_c=3000  blkID=0  aMode=1
  FR_Clutch : autolibcoupling/Disc Clutch  port_config=Simulink  Reff=.091/2  Ndisk=9  Aeff=0.006283185  Peng=320000  Jin=.1  Jout=.1  muk=.088  mus=.089  bin=.001  bout=.001  win_o=pos.xdot_0/veh.TyreLoadedRadius_F  wout_o=pos.xdot_0/veh.TyreLoadedRadius_F  tauC=.01  InitiallyLocked=off  maxAbsSpd=3000  blkID=1
  Gain : Gain  Gain=1/2.71
  Split Torsional Compliance : autolibsharedcoupling/Split Torsional Compliance  port_config=Simulink  cplrMode=Shaft split  extInfo=off  k1=5e4  b1=4e2  omega1_c=1000  theta1_o=0  domega1_o=0  k2=5e4  b2=4e2  omega2_c=1000  theta2_o=0  domega2_o=0  blkID=0  aMode=1
      settings: LibrarySourceBlock=autolibcoupling/Split Torsional Compliance
  Terminator{,1..3} (4 alike) : Terminator
  omega_to_freq_FL : Gain  Gain=98/(2*pi)
  omega_to_freq_FR : Gain  Gain=98/(2*pi)
  Split torsional Compliance Trq : Outport
  Trq_FL : Outport  Port=2
  Trq_FR : Outport  Port=3
  tag scope: Axl_front_Spd=global, FL_G_Spd=global, FL_R_Spd=global, FL_sen=global, FR_G_Spd=global, FR_R_Spd=global, FR_sen=global, Split_tors_FL=global, Split_tors_FR=global
  wires:
  Split Torsional Compliance/1 -> Split torsional Compliance Trq/1
  FR/2 -> Trq_FR/1
  FL/2 -> Trq_FL/1
  FR/1 -> FR_Clutch/3
  FL/1 -> FL_Clutch/3
  FL_Clutch/1 -> Terminator3/1
  FR_Clutch/1 -> Terminator2/1
  FR_Clutch/2 -> Split Torsional Compliance/3
  FL_Clutch/2 -> Split Torsional Compliance/2
  Demux/2 -> [FR_G_Spd], FR/2
  FR_Clutch/3 -> omega_to_freq_FR/1, [FR_R_Spd], FR/1
  Demux/4 -> Terminator1/1
  Demux/3 -> Terminator/1
  Bus Selector/1 -> Demux/1  "<Omega>"
  Veh/1 -> Bus Selector/1
  FL_Clutch/3 -> omega_to_freq_FL/1, [FL_R_Spd], FL/1
  [FR_prs] -> FR_Clutch/1
  [FL_prs] -> FL_Clutch/1
  Split Torsional Compliance/2 -> [Split_tors_FL], FL_Clutch/2  "Front_left_clutch"
  AxlSpd/1 -> Gain/1
  Split Torsional Compliance/3 -> [Split_tors_FR], FR_Clutch/2  "Front_right_clutch"
  omega_to_freq_FL/1 -> [FL_sen]  "FL_freq"
  omega_to_freq_FR/1 -> [FR_sen]  "FR_freq"
  Demux/1 -> [FL_G_Spd], FL/2
  Gain/1 -> [Axl_front_Spd], Split Torsional Compliance/1  "Front axle"

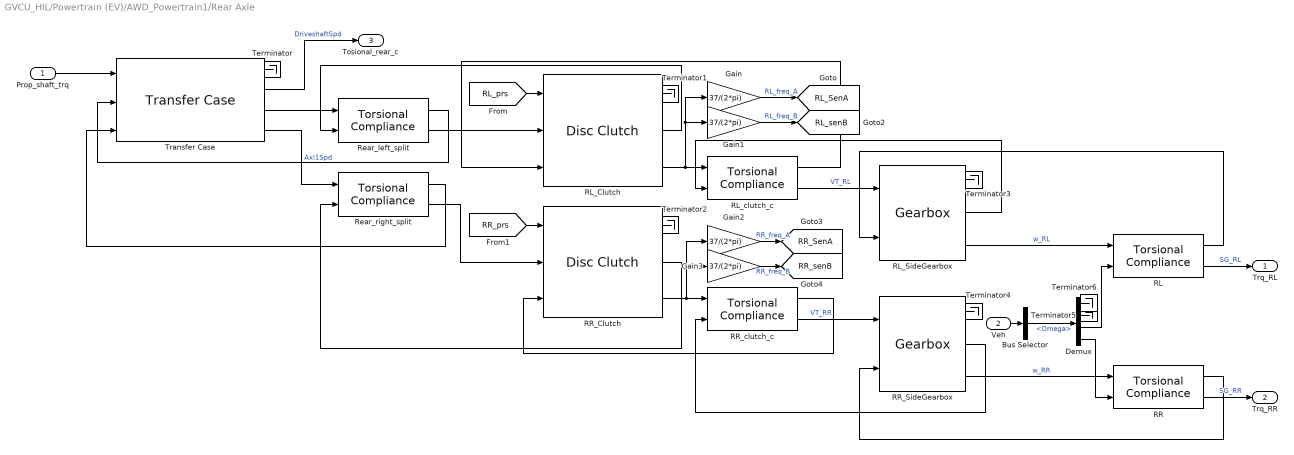
== system GVCU_HIL/Powertrain (EV)/AWD_Powertrain1/Rear Axle ==
  Prop_shaft_trq : Inport
  Veh : Inport  Port=2
  Bus Selector : BusSelector  OutputSignals=Wheels.Omega
  Demux : Demux
  Gain{,1..3} (4 alike) : Gain  Gain=37/(2*pi)
  RL : autolibsharedcoupling/Torsional Compliance  port_config=Simulink  extInfo=off  k=8e4  b=4e2  theta_o=0  domega_o=0  omega_c=3000  blkID=0  aMode=1
  RL_Clutch : autolibcoupling/Disc Clutch  port_config=Simulink  Reff=.091/2  Ndisk=9  Aeff=0.006283185  Peng=320000  Jin=.1  Jout=.1  muk=.088  mus=.089  bin=.001  bout=.001  win_o=pos.xdot_0/veh.TyreLoadedRadius_R*veh.RearSideGear  wout_o=pos.xdot_0/veh.TyreLoadedRadius_R*veh.RearSideGear  tauC=.01  InitiallyLocked=off  maxAbsSpd=3000  blkID=1
  RL_SideGearbox : autolibsharedcoupling/Gearbox  port_config=Simulink  input_config=Torque input - velocity output  DiffEffModelPopup=Constant  InterpMethod=Flat  dirSwitch=on  extTamb=off  N=veh.RearSideGear  J1=.01  J2=.01  b1=.001  b2=.001  theta1_o=0  w1_o=pos.xdot_0/veh.TyreLoadedRadius_R*veh.RearSideGear  eta=1  eta_tbl=reshape([0.64 0.76 0.8 0.81 0.83 0.84 0.84 0.56 0.73 0.78 0.8 0.83 0.84 0.84 0.54 0.71 0.77 0.8 0.82 0.84 0.84 0.53 0.71 0.77 0.8 0.83 0.84 0.84 0.51 0.71 0.77 0.8 0.83 0.84 0.85 0.52 0.7 0.77 0.8 0.83 0.84 0.85 0.51 0.71 0.76 0.79 0.83 0.84 0.85 0.5 0.69 0.76 0.79 0.82 0.84 0.85 0.45 0.68 0.75 0.78 0.82 0.84 0.85 0.43 0.67 0.74 0.78 0.81 0.83 0.84 0.38 0.63 0.71 0.75 0.8 0.82 0.83 0.81 0.86 0.88 0.89 0.89 0.89 0.9 0.77 0.85 0.87 0.88 0.89 0.9 0.9 0.72 0.82 0.86 0.87 0.88 0.89 0.9 0.68 0.8 0.84 0.86 0.88 0.89 0.89 0.67 0.8 0.84 0.86 0.88 0.89 0.9 0.67 0.8 0.84 0.86 0.88 0.89 0.9 0.65 0.8 0.84 0.86 0.88 0.89 0.9 0.64 0.79 0.83 0.86 0.88 0.89 0.9 0.63 0.78 0.83 0.86 0.88 0.89 0.9 0.59 0.76 0.82 0.85 0.87 0.89 0.9 0.53 0.73 0.8 0.83 0.86 0.88 0.89], 7, 11, 2)  Trq_bpts=[25, 50, 75, 100, 150, 200, 250]  omega_bpts=[52.4 78.5 105 131 157 183 209 262 314 419 524]  Temp_bpts=[290 358]  Tamb=297.15  blkID=0  aMode=1
  RL_clutch_c : autolibsharedcoupling/Torsional Compliance  port_config=Simulink  extInfo=off  k=4e4  b=1e2  theta_o=0  domega_o=0  omega_c=3000  blkID=0  aMode=1
  RR : autolibsharedcoupling/Torsional Compliance  port_config=Simulink  extInfo=off  k=8e4  b=4e2  theta_o=0  domega_o=0  omega_c=3000  blkID=0  aMode=1
  RR_Clutch : autolibcoupling/Disc Clutch  port_config=Simulink  Reff=.091/2  Ndisk=9  Aeff=0.006283185  Peng=320000  Jin=.1  Jout=.1  muk=.088  mus=.089  bin=.001  bout=.001  win_o=pos.xdot_0/veh.TyreLoadedRadius_R*veh.RearSideGear  wout_o=pos.xdot_0/veh.TyreLoadedRadius_R*veh.RearSideGear  tauC=.01  InitiallyLocked=off  maxAbsSpd=3000  blkID=1
  RR_SideGearbox : autolibsharedcoupling/Gearbox  port_config=Simulink  input_config=Torque input - velocity output  DiffEffModelPopup=Constant  InterpMethod=Flat  dirSwitch=on  extTamb=off  N=2.38  J1=.01  J2=.01  b1=.001  b2=.001  theta1_o=0  w1_o=pos.xdot_0/veh.TyreLoadedRadius_R*veh.RearSideGear  eta=1  eta_tbl=reshape([0.64 0.76 0.8 0.81 0.83 0.84 0.84 0.56 0.73 0.78 0.8 0.83 0.84 0.84 0.54 0.71 0.77 0.8 0.82 0.84 0.84 0.53 0.71 0.77 0.8 0.83 0.84 0.84 0.51 0.71 0.77 0.8 0.83 0.84 0.85 0.52 0.7 0.77 0.8 0.83 0.84 0.85 0.51 0.71 0.76 0.79 0.83 0.84 0.85 0.5 0.69 0.76 0.79 0.82 0.84 0.85 0.45 0.68 0.75 0.78 0.82 0.84 0.85 0.43 0.67 0.74 0.78 0.81 0.83 0.84 0.38 0.63 0.71 0.75 0.8 0.82 0.83 0.81 0.86 0.88 0.89 0.89 0.89 0.9 0.77 0.85 0.87 0.88 0.89 0.9 0.9 0.72 0.82 0.86 0.87 0.88 0.89 0.9 0.68 0.8 0.84 0.86 0.88 0.89 0.89 0.67 0.8 0.84 0.86 0.88 0.89 0.9 0.67 0.8 0.84 0.86 0.88 0.89 0.9 0.65 0.8 0.84 0.86 0.88 0.89 0.9 0.64 0.79 0.83 0.86 0.88 0.89 0.9 0.63 0.78 0.83 0.86 0.88 0.89 0.9 0.59 0.76 0.82 0.85 0.87 0.89 0.9 0.53 0.73 0.8 0.83 0.86 0.88 0.89], 7, 11, 2)  Trq_bpts=[25, 50, 75, 100, 150, 200, 250]  omega_bpts=[52.4 78.5 105 131 157 183 209 262 314 419 524]  Temp_bpts=[290 358]  Tamb=297.15  blkID=0  aMode=1
  RR_clutch_c : autolibsharedcoupling/Torsional Compliance  port_config=Simulink  extInfo=off  k=4e4  b=1e2  theta_o=0  domega_o=0  omega_c=3000  blkID=0  aMode=1
  Rear_left_split : autolibsharedcoupling/Torsional Compliance  port_config=Simulink  extInfo=off  k=4e4  b=1e2  theta_o=0  domega_o=0  omega_c=3000  blkID=0  aMode=1
  Rear_right_split : autolibsharedcoupling/Torsional Compliance  port_config=Simulink  extInfo=off  k=4e4  b=1e2  theta_o=0  domega_o=0  omega_c=3000  blkID=0  aMode=1
  Terminator{,1..6} (7 alike) : Terminator
  Transfer Case : autolibshareddiff/Transfer Case  DiffEffModelPopup=Constant  InterpMethod=Linear point-slope  extTamb=off  TrqSplitRatioMode=off  SpdLockMode=off  shaftSwitchMask=To the left of center-line  Ndiff=veh.BevelGear_R  Jd=.1  bd=1e-3  Jw1=.1  bw1=1e-3  Jw2=.1  bw2=1e-3  omegaw1o=pos.xdot_0/veh.TyreLoadedRadius_R*veh.RearSideGear  omegaw2o=pos.xdot_0/veh.TyreLoadedRadius_R*veh.RearSideGear  eta=1  eta_tbl=reshape([0.64 0.76 0.8 0.81 0.83 0.84 0.84 0.56 0.73 0.78 0.8 0.83 0.84 0.84 0.54 0.71 0.77 0.8 0.82 0.84 0.84 0.53 0.71 0.77 0.8 0.83 0.84 0.84 0.51 0.71 0.77 0.8 0.83 0.84 0.85 0.52 0.7 0.77 0.8 0.83 0.84 0.85 0.51 0.71 0.76 0.79 0.83 0.84 0.85 0.5 0.69 0.76 0.79 0.82 0.84 0.85 0.45 0.68 0.75 0.78 0.82 0.84 0.85 0.43 0.67 0.74 0.78 0.81 0.83 0.84 0.38 0.63 0.71 0.75 0.8 0.82 0.83 0.81 0.86 0.88 0.89 0.89 0.89 0.9 0.77 0.85 0.87 0.88 0.89 0.9 0.9 0.72 0.82 0.86 0.87 0.88 0.89 0.9 0.68 0.8 0.84 0.86 0.88 0.89 0.89 0.67 0.8 0.84 0.86 0.88 0.89 0.9 0.67 0.8 0.84 0.86 0.88 0.89 0.9 0.65 0.8 0.84 0.86 0.88 0.89 0.9 0.64 0.79 0.83 0.86 0.88 0.89 0.9 0.63 0.78 0.83 0.86 0.88 0.89 0.9 0.59 0.76 0.82 0.85 0.87 0.89 0.9 0.53 0.73 0.8 0.83 0.86 0.88 0.89], 7, 11, 2)  Trq_bpts=[25, 50, 75, 100, 150, 200, 250]  omega_bpts=[52.4 78.5 105 131 157 183 209 262 314 419 524]  Temp_bpts=[290 358]  Tamb=297.15  maxAbsSpd=5e3  aMode=1  TrqSplitRatio=0.5  SpdLock=1
      settings: LibrarySourceBlock=autolibdiff/Transfer Case
  Trq_RL : Outport
  Trq_RR : Outport  Port=2
  Tosional_rear_c : Outport  Port=3
  tag scope: RL_SenA=global, RL_senB=global, RR_SenA=global, RR_senB=global
  wires:
  Transfer Case/2 -> Tosional_rear_c/1  "DriveshaftSpd"
  Demux/4 -> RR/2
  Demux/3 -> RL/2
  Demux/1 -> Terminator6/1
  Bus Selector/1 -> Demux/1  "<Omega>"
  Demux/2 -> Terminator5/1
  Veh/1 -> Bus Selector/1
  RR_SideGearbox/1 -> Terminator4/1
  RR/1 -> RR_SideGearbox/2
  RL/1 -> RL_SideGearbox/2
  RR/2 -> Trq_RR/1  "SG_RR"
  RL/2 -> Trq_RL/1  "SG_RL"
  RR_SideGearbox/3 -> RR/1  "w_RR"
  RR_clutch_c/1 -> RR_Clutch/3
  RR_SideGearbox/2 -> RR_clutch_c/2
  RR_clutch_c/2 -> RR_SideGearbox/1  "VT_RR"
  RR_Clutch/3 -> Gain3/1, Gain2/1, RR_clutch_c/1
  RR_Clutch/2 -> Rear_right_split/2
  RL_Clutch/2 -> Rear_left_split/2
  RL_SideGearbox/1 -> Terminator3/1
  RL_SideGearbox/2 -> RL_clutch_c/2
  RL_SideGearbox/3 -> RL/1  "w_RL"
  RL_clutch_c/2 -> RL_SideGearbox/1  "VT_RL"
  RL_clutch_c/1 -> RL_Clutch/3
  RL_Clutch/3 -> Gain1/1, Gain/1, RL_clutch_c/1
  RR_Clutch/1 -> Terminator2/1
  RL_Clutch/1 -> Terminator1/1
  [RR_prs] -> RR_Clutch/1
  [RL_prs] -> RL_Clutch/1
  Rear_right_split/2 -> RR_Clutch/2
  Rear_right_split/1 -> Transfer Case/3
  Rear_left_split/1 -> Transfer Case/2
  Rear_left_split/2 -> RL_Clutch/2
  Transfer Case/4 -> Rear_right_split/1  "Axl1Spd"
  Transfer Case/3 -> Rear_left_split/1
  Transfer Case/1 -> Terminator/1
  Prop_shaft_trq/1 -> Transfer Case/1
  Gain/1 -> [RL_SenA]  "RL_freq_A"
  Gain1/1 -> [RL_senB]  "RL_freq_B"
  Gain3/1 -> [RR_senB]  "RR_freq_B"
  Gain2/1 -> [RR_SenA]  "RR_freq_A"
